simulink model "DcMotors_PID_Tuning"  (R2018a)
settings: Solver=VariableStepAuto  StartTime=t(1)  StopTime=t(end)  RelTol=1e-3
undefined symbols (not defined in the file): Identified_Model_L, Ts
libraries: simulink x1
settings Model: Creator=peppe  LastModifiedBy=peppe

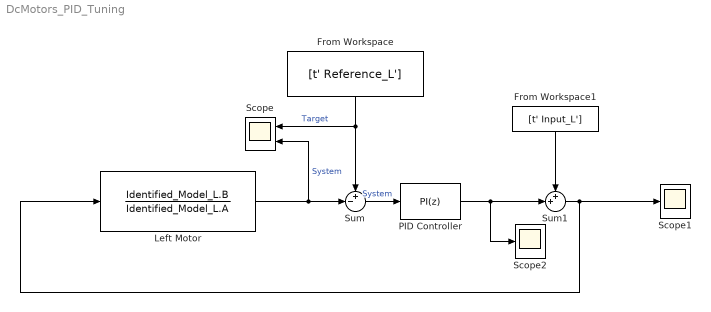
== system DcMotors_PID_Tuning ==
  From Workspace : FromWorkspace  VariableName=[t' Reference_L']  SampleTime=0
  From Workspace1 : FromWorkspace  VariableName=[t' Input_L']  SampleTime=0
  Left Motor : DiscreteTransferFcn  Numerator=Identified_Model_L.B  Denominator=Identified_Model_L.A  SampleTime=Ts
  PID Controller : simulink/Continuous/PID Controller  Controller=PI  TimeDomain=Discrete-time  SampleTime=Ts  IntegratorMethod=Forward Euler  FilterMethod=Forward Euler  Form=Parallel  UseFilter=off  ControllerParametersSource=internal  P=0.165491445149705  I=0.00784747733041369  D=-0.0807109453628274  N=100  InitialConditionSource=internal  InitialConditionForIntegrator=0  InitialConditionForFilter=0  ExternalReset=none  LimitOutput=off  UpperSaturationLimit=2.2  LowerSaturationLimit=-2.2  LinearizeAsGain=on  AntiWindupMode=none  Kb=1  TrackingMode=off  Kt=1  PParamMin=[]  PParamMax=[]  IParamMin=[]  IParamMax=[]  DParamMin=[]  DParamMax=[]  NParamMin=[]  NParamMax=[]  KbParamMin=[]  KbParamMax=[]  KtParamMin=[]  KtParamMax=[]  POutMin=[]  POutMax=[]  IOutMin=[]  IOutMax=[]  DOutMin=[]  DOutMax=[]  NOutMin=[]  NOutMax=[]  KbOutMin=[]  KbOutMax=[]  KtOutMin=[]  KtOutMax=[]  IntegratorOutMin=[]  IntegratorOutMax=[]  FilterOutMin=[]  FilterOutMax=[]  SumOutMin=[]  SumOutMax=[]  SumI1OutMin=[]  SumI1OutMax=[]  SumI2OutMin=[]  SumI2OutMax=[]  SumI3OutMin=[]  SumI3OutMax=[]  SumDOutMin=[]  SumDOutMax=[]  SaturationOutMin=[]  SaturationOutMax=[]  IntegratorContinuousStateAttributes=''  IntegratorStateMustResolveToSignalObject=off  IntegratorRTWStateStorageClass=Auto  FilterContinuousStateAttributes=''  FilterStateMustResolveToSignalObject=off  FilterRTWStateStorageClass=Auto  DifferentiatorICPrevScaledInput=0  DifferentiatorOutMin=[]  DifferentiatorOutMax=[]  FilterDiffOutCoefMin=[]  FilterDiffOutCoefMax=[]  SumDenOutMin=[]  SumDenOutMax=[]  SumNumOutMin=[]  SumNumOutMax=[]  ReciprocalOutMin=[]  ReciprocalOutMax=[]  DivideOutMin=[]  DivideOutMax=[]  TunerSelectOption=Transfer Function Based (PID Tuner App)
  Scope : Scope  NumInputPorts=2
  Scope1 : Scope
  Scope2 : Scope
  Sum : Sum  Inputs=+-|
  Sum1 : Sum  Inputs=++|
  wires:
  Left Motor/1 -> Scope/2, Sum/2  "System"
  Sum/1 -> PID Controller/1  "System"
  From Workspace/1 -> Sum/1, Scope/1  "Target"
  From Workspace1/1 -> Sum1/1
  PID Controller/1 -> Scope2/1, Sum1/2
  Sum1/1 -> Scope1/1, Left Motor/1
